simulink model "Final_EWASP_VC"  (R2022a)
settings: Solver=ode1  StartTime=0.0  StopTime=24*3600  FixedStep=10  RelTol=1e-3
values from neighbouring files (symbols this model uses):
  Aux_Threshold = 52    [Setup_Code_EWASP_VC.m]
  buildingAge = 2005    [Setup_Code_EWASP_VC.m]
  ceilingHeight = 2.4    [Setup_Code_EWASP_VC.m]
  conductiveHconnectMatrix = [ ... (first row only)    [Setup_Code_EWASP_VC.m]
  cRoofGreen = 100000    [Setup_Code_EWASP_VC.m]
  Defrost_After_Time = 30    [Setup_Code_EWASP_VC.m]
  DHWDemandProfile = occFreegainHotwaterElecTestPassiveOcc3(:,3)    [Setup_Code_EWASP_VC.m]
  Elec_Max = Elec_Max*(30/24.2)    [Setup_Code_EWASP_VC.m]
  Elec_Mid = Elec_Mid*(30/24.2)    [Setup_Code_EWASP_VC.m]
  Elec_Min = Elec_Min*(30/24.2)    [Setup_Code_EWASP_VC.m]
  ElecDemandProfile = occFreegainHotwaterElecTestPassiveOcc3(:,4)    [Setup_Code_EWASP_VC.m]
  ElecFixed = [Elec_Max(6,2) Elec_Max(6,4) Elec_Max(6,6) Elec_Max(6,7) ... (first row only)    [Setup_Code_EWASP_VC.m]
  floorOrCeilingArea = floorOrCeilingArea*1.15    [Setup_Code_EWASP_VC.m]
  forceCold = 0    [Setup_Code_EWASP_VC.m]
  freegain = occFreegainHotwaterElecTestPassiveOcc3(:,2)-max(occupancy)*25    [Setup_Code_EWASP_VC.m]
  furnitureModelOn = 1    [Setup_Code_EWASP_VC.m]
  Heat_Max = Heat_Max*(30/24.2)    [Setup_Code_EWASP_VC.m]
  Heat_Mid = Heat_Mid*(30/24.2)    [Setup_Code_EWASP_VC.m]
  Heat_Min = Heat_Min*(30/24.2)    [Setup_Code_EWASP_VC.m]
  HeatFixed = [Heat_Max(6,2) Heat_Max(6,4) Heat_Max(6,6) Heat_Max(6,7) ... (first row only)    [Setup_Code_EWASP_VC.m]
  HeatingOnProfile = repmat(HeatingOnProfile,365,1)    [Setup_Code_EWASP_VC.m]
  HEX_ReturnLowerLimit = 52.5    [Setup_Code_EWASP_VC.m]
  HEX_ReturnUpperLimit = 55    [Setup_Code_EWASP_VC.m]
  LeakMultiplier = 1+(2*(rand()-0.5)/10)    [Setup_Code_EWASP_VC.m]
  loopCap = 15    [Setup_Code_EWASP_VC.m]
  maxOcc = max(occupancyProfile)    [Setup_Code_EWASP_VC.m]
  NESW_wallArea = max(NESW_Lengths*ceilingHeight-NESW_Windows,0)    [Setup_Code_EWASP_VC.m]
  NESW_Windows = [ ... (first row only)    [Setup_Code_EWASP_VC.m]
  numRooms = roomCount    [Setup_Code_EWASP_VC.m]
  offsetDays = 0    [Setup_Code_EWASP_VC.m]
  pumpChoice = pumpChoices(MinIndex,1)    [Setup_Code_EWASP_VC.m]
  pumpRamp = 180    [Setup_Code_EWASP_VC.m]
  ReturnLowerLimit = 37.5    [Setup_Code_EWASP_VC.m]
  ReturnUpperLimit = 40    [Setup_Code_EWASP_VC.m]
  RoofIrradiance = Flat_NS_EW_RoofIrradiance(:,1)    [Setup_Code_EWASP_VC.m]
  roofStartTemp = ones(11,1)*20    [Setup_Code_EWASP_VC.m]
  rooftype = 0    [Setup_Code_EWASP_VC.m]
  RoomDataMatrix = [zeros(1,12);ones(1,12)*wallDensity;zeros(1,12);ones(1,12)*wallU;ones(1,12)*windowU;ones(1,12)*floorU;ones(1,12)*ceilingU;zeros(1,12);windowArea, 0;floorOrCeilingArea;zeros(1,12);floorOrCeilingArea*ceilingHeight]    [Setup_Code_EWASP_VC.m]
  roomVol = roomVol*1.15    [Setup_Code_EWASP_VC.m]
  slabStartTemp = (GroundTempTimeSeries(offsetDays*1440+1,1)+thermostatSetting)/2    [Setup_Code_EWASP_VC.m]
  SlackRequest = zeros(1440,1)    [Setup_Code_EWASP_VC.m]
  SolarThermalExists = 0    [Setup_Code_EWASP_VC.m]
  SourceFixed = HeatFixed-ElecFixed    [Setup_Code_EWASP_VC.m]
  StateSeries = StateSeriesGenerator(22,7,1)    [Setup_Code_EWASP_VC.m]
  Tank_Lower_Temp = 49.5    [Setup_Code_EWASP_VC.m]
  Tank_Upper_Temp = 52    [Setup_Code_EWASP_VC.m]
  Tank_Volume_m3 = 0.15    [Setup_Code_EWASP_VC.m]
  TankHeatHour = randi([1 5])-1    [Setup_Code_EWASP_VC.m]
  thermostatSetting = 20.0    (= 20)    [Setup_Code_EWASP_VC.m]
  upDown = [0;0;0;0;1;1;1;1;1;1;1]    [Setup_Code_EWASP_VC.m]
  variableASHP = 1    [Setup_Code_EWASP_VC.m]
  wallStartTempExt = thermostatSetting*(0.266+0.00215*outdoorStartTemp+0.018*wallU+0.00113*outdoorStartTemp*wallU+0.0068*wallU^2)    [Setup_Code_EWASP_VC.m]
undefined symbols (not defined in the file or in its folder): a, ceilingU, condUDMatrix, convUDMatrix, deltaPEXPANDED_E, deltaPEXPANDED_E2, deltaPEXPANDED_N, deltaPEXPANDED_N2, deltaPEXPANDED_S, deltaPEXPANDED_S2, deltaPEXPANDED_W, deltaPEXPANDED_W2, DesiredDHWTemp, DesiredFlowTempVsInOutDeltaTemp, DiffuseHorizontal, DiscIntNeverNeededParam, DNI, dwnAndConcrete, DWORK_A_HX, DWORK_CHK_FLU, DWORK_CP_NODE, DWORK_DH, DWORK_FLUID, DWORK_HCON, DWORK_LOSS, DWORK_MDOTDOWN, DWORK_MDOTIN, DWORK_MDOTUP, DWORK_MIX, DWORK_PRESS, DWORK_QDOTIN, DWORK_RHO_NODE, DWORK_TIN, DWORK_TS_OLD, DWORK_V_NODE, GroundTempTimeSeries, HCM, HCM2, HCM_closed, HCM_closed2, intermediateU, IsTop, massFlowMatrix, neighbourMatrix, numericalRoomUse, RadiatorMatrix, room2roomflowmatrix_E, room2roomflowmatrix_E2, room2roomflowmatrix_N, room2roomflowmatrix_N2, room2roomflowmatrix_S, room2roomflowmatrix_S2, room2roomflowmatrix_W, room2roomflowmatrix_W2, StateAirInEXPANDED_E, StateAirInEXPANDED_E2, StateAirInEXPANDED_N, StateAirInEXPANDED_N2, StateAirInEXPANDED_S, StateAirInEXPANDED_S2 ... (+23)
libraries: simulink x6, dspsigops x4, dspmtrx3 x4, carnot x3, spsEdgeDetectorLib x2, dspstat3 x2, powerlib_meascontrol x1, simulink_extras x1
(part 4 of 27)

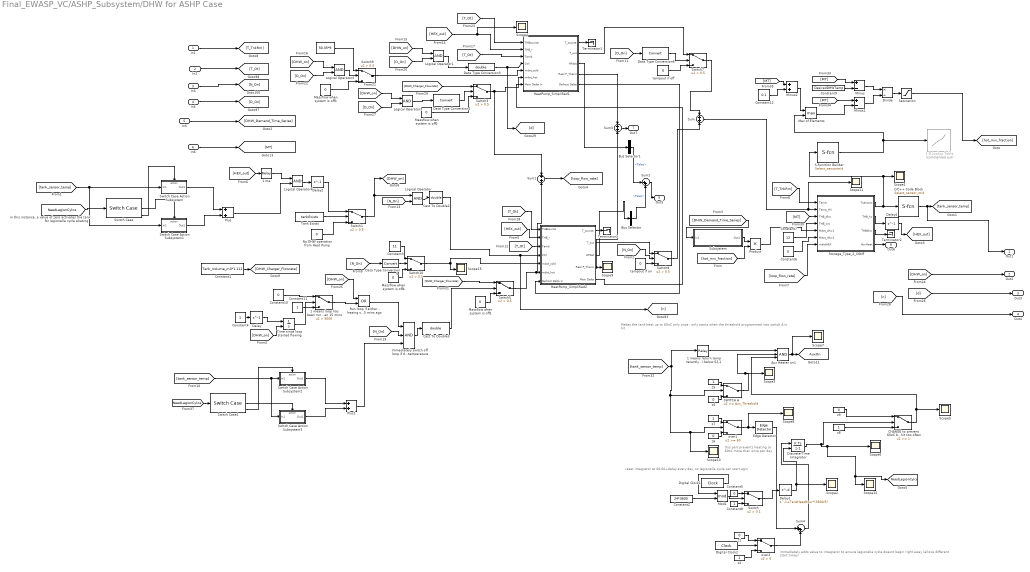
== system Final_EWASP_VC/ASHP_Subsystem/DHW for ASHP Case ==
  note: immediately adds value to integrator to ensure legionella cycle doesnt begin right away (allows different start times)
  note: this part prevents heating
      | to 60oC more than once per
      | day
  note: reset integrator at 00:00+delay every day,
      | so legionella cycle can start agin
  note: Makes the tank heat up to 60oC only once - only starts when the threshold programmed into switch A is hit
  In1 : Inport
  In2 : Inport  Port=2
  In3 : Inport  Port=3
  In4 : Inport  Port=4
  In5 : Inport  Port=5
  In6 : Inport  Port=6
  " " : Constant  Value=50.35*9  OutDataTypeStr=double
  1 me : Relay  OnSwitchValue=HEX_ReturnUpperLimit  OffSwitchValue=HEX_ReturnLowerLimit  OnOutputValue=0  OffOutputValue=1  OutDataTypeStr=boolean
  1 means loop has been running for less than 15 mins : Switch  Criteria=u2 > Threshold  Threshold=9000  SaturateOnIntegerOverflow=off  InputSameDT=off
  1 means return temp recently fell below 52.1 : Relay  OnSwitchValue=61  OffSwitchValue=59  OnOutputValue=0  OffOutputValue=1  OutDataTypeStr=boolean
  1-D Lookup Table : Lookup_n-D  Commented=on  NumberOfTableDimensions=1  BreakpointsForDimension1=[0:100]  Table="[1 1\t1\t1\t1\t1\t1\t1\t1\t1\t1\t1\t1\t1\t1\t1\t1\t1\t1\t1\t1\t1\t1\t1\t1\t1\t1\t1\t1\t1\t1\t1\t1\t1\t1\t1\t1\t1\t1\t1\t1\t1\t1\t1\t1\t1\t1\t1\t1\t1\t1\t1\t0.975000000000000\t0.951219512195122\t0.928571428571429\t0.906976744186047\t0.886363636363636\t0.866666666666667\t0.847826086956522\t0.829787234042553\t0.812500000000000\t0.795918367346939\t0.780000000000000\t0.764705882352941\t0.750000000000000\t0.735849056603774\t0.722222222222222\t0.709090909090909\t0.696428571428571\t0.684210526315790\t0.672413793103448\t0.661016949152542\t0.650000000000000\t0.639344262295082\t0.629032258064516\t0.619047619047619\t0.609375000000000\t0.600000000000000\t0.590909090909091\t0.582089552238806\t0.573529411764706\t0.565217391304348\t0.557142857142857\t0.549295774647887\t0.541666666666667\t0.534246575342466\t0.527027027027027\t0.520000000000000\t0.513157894736842\t0.506493506493506\t0.500000000000000\t0.493670886075949\t0.487500000000000\t0.481481481481481\t0.475609756097561\t0.469879518072289\t0.464285714285714\t0.458823529411765\t0.453488372093023\t0.448275862068966\t0.443181818181818]"  InternalRulePriority=Speed  RndMeth=Simplest
  Aux Heater on1 : Logic  Inputs=3  AllPortsSameDT=off  OutDataTypeStr=boolean
  Bus Selector : BusSelector  OutputSignals=Pelec
  Bus Selector1 : BusSelector  OutputSignals=Pelec
  C/C++ Code Block : S-Function  InitFcn=try, set_param(gcb,'FunctionName','Select_sensor_mid'), end  FunctionName=Select_sensor_mid  SFunctionModules=Select_sensor_mid_wrapper  SFunctionDeploymentMode=off  EnableBusSupport=off  mask(S-Function Builder){}
      mask help: Simulink:masks:SFunctionBuilder_MD
      mask init:
      | val = [[.9  0.75 0.75 1 1 .9 .9 1]',[1 1 0.75 0.75 .9 .9 1 .9]'];try , sys = get_param(gcb,'SfunBuilderFcnName');if isempty(sys), sys = get_param(gcb,'FunctionName'); end,catch, sys = get_param(gcb,'FunctionName'); end
      settings: CopyFcn=set_param(gcbh,'LinkStatus','none')  PreSaveFcn=try, set_param(gcb,'FunctionName','Select_sensor_mid'), end  OpenFcn=sfunctionwizard(gcbh)
      mask Display: plot(val(:,1),val(:,2)),disp(sys), port_label('input',1,'u0'), port_label('output',1,'y0')
  CHANGE to prevent 60oC being hit too often : Switch  Threshold=1  SaturateOnIntegerOverflow=off  InputSameDT=off
  Cast To Double2 : DataTypeConversion  OutDataTypeStr=double  SaturateOnIntegerOverflow=off  RndMeth=Floor
  Cast To Double3 : DataTypeConversion  OutDataTypeStr=double  SaturateOnIntegerOverflow=off  RndMeth=Floor
  Constant1 : Constant  Value=Tank_Volume_m3*1.111
  Constant10 : Constant  Value=0
  Constant11 : Constant
  Constant12 : Constant  Value=0.1
  Constant2 : Constant  Value=24*3600
  Constant3 : Constant  Value=11
  Constant4 : Constant
  Constant5 : Constant  Value=0
  Constant6 : Constant  Value=0
  Constant7 : Constant  Value=12
  Constant8 : Constant
  Constant9 : Constant  Value=DesiredDHWTemp
  Data Type Conversion3 : DataTypeConversion  OutDataTypeStr=double  SaturateOnIntegerOverflow=off  RndMeth=Floor
  Data Type Conversion4 : DataTypeConversion  RndMeth=Round  SaturateOnIntegerOverflow=off
  Data Type Conversion5 : DataTypeConversion  RndMeth=Round  SaturateOnIntegerOverflow=off
  Data Type Conversion6 : DataTypeConversion  RndMeth=Round  SaturateOnIntegerOverflow=off
  Delay : Delay  DelayLength=1  InitialCondition=0
  Delay1 : Delay  DelayLength=1+TankHeatHour*(3600/5)  InitialCondition=0
  Delay2 : Delay  DelayLength=1  InitialCondition=1
  Delay4 : Delay  DelayLength=1  InitialCondition=0
  Digital Clock1 : DigitalClock  SampleTime=10
  Digital Clock2 : DigitalClock  SampleTime=10
  Discrete-Time Integrator : DiscreteIntegrator  ExternalReset=rising  SampleTime=-1  OutDataTypeStr=double  ICPrevOutput=DiscIntNeverNeededParam  ICPrevScaledInput=DiscIntNeverNeededParam
  Divide : Product  Inputs=*/
  Edge Detector : spsEdgeDetectorLib/Edge Detector  model=Rising  ic=0  Ts=-1
      settings: SourceProductBaseCode=PS
  HeatPump_Simplified1 : Subsystem  AncestorBlock=carnot/Source/Heat_Pump/HeatPump  mask(heat pump){Tcin=[-5 15], Thout=[35 45 55 60], Qdotc=[-6125 -6125 -6125 -6125;-6125 -6125 -6125 -6125], Qdoth=[-3000*a -3000*a -3000*a -3000*a;-3000*a -3000*a -3000*a -3000*a], Pel=[1625*a 1625*a 1625*a 1625*a;1625*a 1625*a 1625*a 1625*a], caph=10*4180, capc=inf, UA=0, linc=10, quac=10, linh=10, quah=10}
      mask prompts: Tcin "inlet source temperature vector (°C)"; Thout "outlet load temperature vector (°C)"; Qdotc "source power matrix (W)"; Qdoth "heating power matrix (W)"; Pel "electric power matrix (W)"; caph "thermal capacity hot loop [J/K]"; capc "thermal capacity cold loop [J/K]"; UA "heat loss coefficient [W/K]"; linc "Cold side linear massflow dependant pressure drop in [Pa*s/kg]"; quac "Cold side quadratic massflow dependant pressure drop hot side in [Pa*s²/kg]"; linh "Hot side linear massflow dependant pressure drop in [Pa*s/kg]"; quah "Hot side quadratic massflow dependant pressure drop hot side in [Pa*s²/kg]"
      mask help:
      | Linearized heat pump model. Uses measured data according to EN 14511 as input.
      | heating power: Qdot_h = K1*Tcold_in + K2*Thot_out + K3
      | electric power: Pel = K4*Tcold_in + K5*Thot_out + K6
      | source power: Qdot_c = -K7*Tcold_in - K8*Thot_out - K9
      | differential equation: cap*dTh/dt = Qdot + mdot*cp*(T_in-T) + UA*(Tamb-T)
      | with: cap = mass * heat_capactiy
      | See hp_param.m for the parameters K1 to K9.
      | Literature: Schwamberger, K.: Fortschrittsberichete VDI, Nr. 263, 1991
      mask init:
      | % Matrix construction for hp_param
      | A = reshape(Qdoth',numel(Qdoth),1);
      | A = [A reshape(Qdotc',numel(Qdotc),1)];
      | A = [A reshape(Pel',numel(Pel),1)];
      | Thout_temp = [];
      | Tcin_temp = [];
      | for i=1:numel(Tcin)
      |     for j=1:numel(Thout)
      |         Tcin_temp = [Tcin_temp ; Tcin(i)];
      |     end
      |     Thout_temp = [Thout_temp ; Thout'];
      | end
      | A = [A Tcin_temp Thout_temp];
      | 
      | K = hp_param(A);
      | caph = max(1,caph);
      | capc = max(1,capc);
      mask Help: web(fullfile(path_carnot('help'),'heatpump.html'),'-helpbrowser')
      mask DialogControl ParameterTabVar0 Prompt: HP Caracteristic
      mask DialogControl ParameterTabVar01 Prompt: Thermal
      mask DialogControl ParameterTabVar012 Prompt: Hydraulic
      mask Display: plot(-20,-10,120,110,[10,20,40,60,80,90,90,80,60,40,20,10,10],[60,80,90,90,80,60,40,20,10,10,20,40,60],[40,20],[90,20],[60,80],[90,20],[50,50],[30,50],[60,40],[40,40],[57,43],[33,46],[44,57],[34,46])
  HeatPump_Simplified2 : Subsystem  AncestorBlock=carnot/Source/Heat_Pump/HeatPump  mask(heat pump){Tcin=[-5 5 12], Thout=[35 45 55 60], Qdotc=[4400*a-2000*a 4200*a-2000*a 3200*a-2000*a 1800*a-2000*a;5800*a-2100*a 5500*a-2100*a 4200*a-2100*a 2800*a-2100*a;8400*a-2200*a 7200*a-2200*a 5500*a-2200*a 3300*a-2200*a], Qdoth=[4400*a 4200*a 3200*a 1800*a;5800*a 5500*a 4200*a 2800*a;8400*a 7200*a 5500*a 3300*a], Pel=[2000*a 2000*a 2000*a 2000*a;2100*a 2100*a 2100*a 2100*a;2200*a 2200*a 2200*a 2200*a], caph=10*4180, capc=inf, UA=2, linc=10, quac=10, linh=10, quah=10}
      mask prompts: Tcin "inlet source temperature vector (°C)"; Thout "outlet load temperature vector (°C)"; Qdotc "source power matrix (W)"; Qdoth "heating power matrix (W)"; Pel "electric power matrix (W)"; caph "thermal capacity hot loop [J/K]"; capc "thermal capacity cold loop [J/K]"; UA "heat loss coefficient [W/K]"; linc "Cold side linear massflow dependant pressure drop in [Pa*s/kg]"; quac "Cold side quadratic massflow dependant pressure drop hot side in [Pa*s²/kg]"; linh "Hot side linear massflow dependant pressure drop in [Pa*s/kg]"; quah "Hot side quadratic massflow dependant pressure drop hot side in [Pa*s²/kg]"
      mask help:
      | Linearized heat pump model. Uses measured data according to EN 14511 as input.
      | heating power: Qdot_h = K1*Tcold_in + K2*Thot_out + K3
      | electric power: Pel = K4*Tcold_in + K5*Thot_out + K6
      | source power: Qdot_c = -K7*Tcold_in - K8*Thot_out - K9
      | differential equation: cap*dTh/dt = Qdot + mdot*cp*(T_in-T) + UA*(Tamb-T)
      | with: cap = mass * heat_capactiy
      | See hp_param.m for the parameters K1 to K9.
      | Literature: Schwamberger, K.: Fortschrittsberichete VDI, Nr. 263, 1991
      mask init: same as Final_EWASP_VC/ASHP_Subsystem/DHW for ASHP Case/HeatPump_Simplified1
      mask Help: web(fullfile(path_carnot('help'),'heatpump.html'),'-helpbrowser')
      mask DialogControl ParameterTabVar0 Prompt: HP Caracteristic
      mask DialogControl ParameterTabVar01 Prompt: Thermal
      mask DialogControl ParameterTabVar012 Prompt: Hydraulic
      mask Display: plot(-20,-10,120,110,[10,20,40,60,80,90,90,80,60,40,20,10,10],[60,80,90,90,80,60,40,20,10,10,20,40,60],[40,20],[90,20],[60,80],[90,20],[50,50],[30,50],[60,40],[40,40],[57,43],[33,46],[44,57],[34,46])
  "Immediately switch off loop if defrost is required, or if tank reaches temperature" : Logic  Inputs=3  AllPortsSameDT=off  OutDataTypeStr=boolean
  Logical Operator{,1..4} (5 alike) : Logic  AllPortsSameDT=off  OutDataTypeStr=boolean
  Massflow when system is off{1..4} (4 alike) : Constant  Value=0
  Max of Elements : MinMax  Function=max  Inputs=2
  Minus : Sum  Inputs=+-
  Minus1 : Sum  Inputs=+-
  Minus2 : Sum  Inputs=2
  Mod1 : Math  Operator=mod  SignedPower=on
  No DHW operation from Heat Pump : Constant  Value=0
  Plus : Sum
  Plus1 : Sum
  Product : Product
  "Run loop if either - heaing system is on, heating system was activated less than 15 mins ago" : Logic  Operator=OR  AllPortsSameDT=off  OutDataTypeStr=boolean
  S-Function Builder : S-Function  InitFcn=try, set_param(gcb,'FunctionName','Select_sensor'), end  FunctionName=Select_sensormid  SFunctionModules=Select_sensor_wrapper  SFunctionDeploymentMode=off  EnableBusSupport=off  mask(S-Function Builder){}
      mask help: Simulink:masks:SFunctionBuilder_MD
      mask init: same as Final_EWASP_VC/ASHP_Subsystem/DHW for ASHP Case/C/C++ Code Block
      settings: CopyFcn=set_param(gcbh,'LinkStatus','none')  PreSaveFcn=try, set_param(gcb,'FunctionName','Select_sensormid'), end  OpenFcn=sfunctionwizard(gcbh)
      mask Display: plot(val(:,1),val(:,2)),disp(sys), port_label('input',1,'u0'), port_label('output',1,'y0')
  SWITCH A : Switch  Threshold=Aux_Threshold  SaturateOnIntegerOverflow=off  InputSameDT=off
  Saturation : Saturate  UpperLimit=1  LowerLimit=0
  Scope{1..12,15} (13 alike) : Scope
  Storage_Type_2_CONF : Subsystem  AncestorBlock=carnot/Storage/Thermal/Storage_Type_2_CONF  mask(Storage for hot water production){t0=52.1, hgt=1.5279, stgtype=2, tini=[52.1 52.1 52.1 52.1 52.1 52.1 52.1 52.1 52.1 52.1], mpts=[1 2 3 4 5 6 7 8 9 10], PathName=fullfile(pwd,'TankVolTemp'), FileName='<user defined>', userPath=on, userParam=on, uwall=0.235, ubot=0.235, utop=0.235, axcond=0.235, volume=Tank_Volume_m3, dia=((4/(3*3.142))*Tank_Volume_m3)^(1/3), standing=standing cylinder, nodes=10, mpoints=10, Tsensor=[0.1:0.1:0.9], hx1inlet=0.45, hx1outlet=0, hx1dia=0.03, hx1uac=500, hx1uam=0.15, hx1uat=0.6, hx1dpqua=20, hx1dplin=20, pipe1inlet=0, pipe1outlet=1, pipe1dia=0.03, pipe2inlet=0.6, pipe2outlet=1, pipe2dia=0.03}
      mask prompts: t0 "Initial temperature (vector or scalar) in °C"; hgt "Height of storage in m"; stgtype "Storage Type (0..5)"; tini "Start temperatures of nodes in °C"; mpts "Index to measured nodes"; PathName "Path"; FileName "Parameter set"; userPath "Edit path and name of parameter set"; userParam "User defined parameters"; uwall "Heat transfer coefficient to ambient [W/m²K]"; ubot "Heat transfer coefficient to ambient bottom [W/m²K]"; utop "Heat transfer coefficient to ambient top [W/m²K]"; axcond "Effective thermal conductivity [W/m/K]"; volume "Volume [m³]"; dia "Diameter [m]"; standing "Position"; nodes "Number of nodes"; mpoints "Number of node temperatures (for display)"; Tsensor "Temperature sensor position (0..1, 0 = bottom, 1 = top)"; hx1inlet "relative height of inlet"; hx1outlet "relative height of outlet"; hx1dia "Diameter of HX pipe [m]"; hx1uac "uac: heat transfer coefficient [W/K /(kg/s) /(°C)]"; hx1uam "uam: massflow dependent heat transfer [-]"; hx1uat "uat: temperature difference dependent heat transfer [-]"; hx1dpqua "pressure drop quadratic in mdot [Pa*s²/kg²]"; hx1dplin "pressure drop linear in mdot [Pa*s/kg]"; pipe1inlet "relative height of inlet, range from 0 (= bottom) to 1 (= top)"; pipe1outlet "relative height of outlet, range from 0 (= bottom) to 1 (= top)"; pipe1dia "Diameter of pipe in m"; pipe2inlet "relative height of inlet, range from 0 (= bottom) to 1 (= top)"; pipe2outlet "relative height of outlet, range from 0 (= bottom) to 1 (= top)"; pipe2dia "Diameter of pipe in m"
      mask help:
      | Storage for hot water production (domestic hot water cylinder). The storage model has the following components (with their typical position):
      | - one charging heat exchanger (lower part)
      | - one pipe connection for the hot water (total height)
      | - one pipe connection for the hot water circulation (upper part )
      mask init:
      | %[ok, param] = CarnotCallbacks_StorageConf('SetParam',stgtype,gcbh,PathName,FileName);
      mask Help: web(fullfile(path_carnot('help'),'Storage_Type_N.html'),'-helpbrowser')
      mask TypeOptions hgt: HX_EN12977_1/hgt | Pipe_Connection_1/hgt | Pipe_Connection_2/hgt
      mask TypeOptions stgtype: CreateSdat/stgtype
      mask TypeOptions tini: sfun_storageTnodesjh/tini
      mask TypeOptions mpts: select_T/Indices
      mask Callback userPath: [ok, param] = CarnotCallbacks_StorageConf('UserEdit',2,gcbh);
      mask Callback userParam: [ok, param] = CarnotCallbacks_StorageConf('UserEdit',2,gcbh);
      mask TypeOptions uwall: sfun_storageTnodesjh/uloss
      mask TypeOptions ubot: sfun_storageTnodesjh/ubot
      mask TypeOptions utop: sfun_storageTnodesjh/utop
      mask TypeOptions axcond: sfun_storageTnodesjh/cond
      mask TypeOptions volume: sfun_storageTnodesjh/volume
      mask TypeOptions dia: sfun_storageTnodesjh/dia
      mask TypeOptions standing: sfun_storageTnodesjh/standing
      mask TypeOptions nodes: sfun_storageTnodesjh/nodes | select_T/InputPortWidth | HX_EN12977_1/nodes | HX_EN12977_2/nodes | HX_EN12977_3/nodes | Pipe_Connection_1/nodes | Pipe_Connection_2/nodes | Pipe_Connection_3/nodes
      mask TypeOptions Tsensor: T_Sensor_Surface/pos
      mask TypeOptions hx1inlet: HX_EN12977_1/h_in
      mask TypeOptions hx1outlet: HX_EN12977_1/h_out
      mask TypeOptions hx1dia: HX_EN12977_1/dia
      mask TypeOptions hx1uac: HX_EN12977_1/ua0
      mask TypeOptions hx1uam: HX_EN12977_1/uam
      mask TypeOptions hx1uat: HX_EN12977_1/uat
      mask TypeOptions hx1dpqua: HX_EN12977_1/dpqua
      mask TypeOptions hx1dplin: HX_EN12977_1/dplin
      mask TypeOptions pipe1inlet: Pipe_Connection_1/h_in
      mask TypeOptions pipe1outlet: Pipe_Connection_1/h_out
      mask TypeOptions pipe1dia: Pipe_Connection_1/dia
      mask TypeOptions pipe2inlet: Pipe_Connection_2/h_in
      mask TypeOptions pipe2outlet: Pipe_Connection_2/h_out
      mask TypeOptions pipe2dia: Pipe_Connection_2/dia
      mask DialogControl Container14 Prompt: Infos
      mask DialogControl ParameterGroupVar Prompt: Picking a parameter set
      mask DialogControl Control3 Prompt: Carnot public data
      mask DialogControl Control3 Callback: [ok, file] = CarnotCallbacks_StorageConf('GetFilename',2,gcbh,'public');
      mask DialogControl Control4 Prompt: Carnot internal data
      mask DialogControl Control4 Callback: [ok, file] = CarnotCallbacks_StorageConf('GetFilename',2,gcbh,'internal');
      mask DialogControl Control2 Prompt: Selected path
      mask DialogControl Control2 Callback: [ok, file] = CarnotCallbacks_StorageConf('GetFilename',2,gcbh,'selected');
      mask DialogControl Container4 Prompt: Parameter values
      mask DialogControl Container6 Prompt: Storage
      mask DialogControl Container8 Prompt: Connections
      mask DialogControl Container11 Prompt: Heat exchanger
      mask DialogControl Container9 Prompt: Discharging pipe
      mask DialogControl Container12 Prompt: Circulation pipe
      mask DialogControl Control6 Prompt: Save in Carnot internal data
      mask DialogControl Control6 Callback: [ok, param] = CarnotCallbacks_StorageConf('SaveFilename',2,gcbh,'internal','STG');
      mask DialogControl Control5 Prompt: Save in selected path
      mask DialogControl Control5 Callback: [ok, param] = CarnotCallbacks_StorageConf('SaveFilename',2,gcbh,'selected','STG');
      mask Display:
      | % user defined picture file
      | namestr = ['Storage_Type_', num2str(get_param(gcb,'stgtype'))];
      | picfile = fullfile(path_carnot('intlibsl'), 'Storage','Thermal', ...
      |     namestr,'parameter_set', [namestr, '.jpg']);
      | 
      | % show public picture
      | plot([36,36,40,50,54,54,50,40,36]/90,...
      |     [90,50,45,45,50,90,93,93,90]/100,[36,51,44,51,36]/90,...
      |     [50,50,55,60,60]/100)
      | set_param(gcb, 'BackgroundColor', 'Red')
      | 
      | % show internal picture if defined
      | if  ~BlockIsInCarnotLibrary       % if not located in library
      |     if exist(picfile, 'file')
      |         image(imread(picfile), [0.25, 0, 0.45, 1])
      |         set_param(gcb, 'BackgroundColor', 'White')
      |     end
      | end
  Subsystem : Subsystem
      mask Display:
      | disp('Minute to \n Second Res')
      | port_label('input', 1, 'min res')
      | port_label('output', 1, 'sec res')
  Sum : Sum
  Sum1 : Sum
  Sum2 : Sum  Inputs=|++
  Sum3 : Sum
  Sum4 : Sum  Inputs=|++
  Switch : Switch  Criteria=u2 > Threshold  Threshold=0.1  SaturateOnIntegerOverflow=off  InputSameDT=off
  Switch Case : SwitchCase  CaseConditions={1,0}
  Switch Case Action Subsystem : Subsystem  TreatAsAtomicUnit=on
  Switch Case Action Subsystem1 : Subsystem  TreatAsAtomicUnit=on
  Switch Case Action Subsystem2 : Subsystem  TreatAsAtomicUnit=on
  Switch Case Action Subsystem3 : Subsystem  TreatAsAtomicUnit=on
  Switch Case1 : SwitchCase  CaseConditions={1,0}
  Switch{1,3,5,7..10} (7 alike) : Switch  Criteria=u2 > Threshold  Threshold=0.5  SaturateOnIntegerOverflow=off  InputSameDT=off
  Tank Exists : Constant  Value=tankExists
  Terminator1 : Terminator
  Terminator2 : Terminator
  Terminator3 : Terminator
  Time since loop started flowing : Integrator  ExternalReset=rising
  over1 : Switch  Threshold=60  SaturateOnIntegerOverflow=off  InputSameDT=off
  over2 : Switch  Criteria=u2 > Threshold  SaturateOnIntegerOverflow=off  InputSameDT=off
  tempout if off : Constant  Value=0
  tempout if on : Constant  Value=0
  z{1,4,6,9} (4 alike) : Constant  Value=0
  z{2,5,7..8} (4 alike) : Constant
  Out1 : Outport  VectorParamsAs1DForOutWhenUnconnected=off
  Out2 : Outport  Port=2  VectorParamsAs1DForOutWhenUnconnected=off
  Out3 : Outport  Port=3  VectorParamsAs1DForOutWhenUnconnected=off
  Out4 : Outport  Port=4  VectorParamsAs1DForOutWhenUnconnected=off
  Out5 : Outport  Port=5  VectorParamsAs1DForOutWhenUnconnected=off
  Out6 : Outport  Port=6  VectorParamsAs1DForOutWhenUnconnected=off
  Out7 : Outport  Port=7  VectorParamsAs1DForOutWhenUnconnected=off
  tag scope: AuxOn=global, NeedLegionCylce=global
  wires:
  [T_Ot] -> HeatPump_Simplified2/3(Tamb)
  [DHW_Charger_Flowrate] -> Switch5/1
  [HEX_out] -> Scope4/1, HeatPump_Simplified1/2(THB_r)
  [T_Ot] -> HeatPump_Simplified1/3(Tamb)
  In4/1 -> [D_On]
  Logical Operator1/1 -> Data Type Conversion3/1
  [T_TnkRm] -> Storage_Type_2_CONF/1(Tamb)
  Sum1/1 -> [loop_flow_rate]
  Product/1 -> Storage_Type_2_CONF/5(Mdot_dhw1)
  "Immediately switch off loop if defrost is required, or if tank reaches temperature"/1 -> Cast To Double3/1
  [DHW_on] -> "Run loop if either - heaing system is on, heating system was activated less than 15 mins ago"/1
  Constant11/1 -> 1 means loop has been running for less than 15 mins/3
  Switch8/1 -> Sum/2
  Constant7/1 -> Storage_Type_2_CONF/4(THB_circ)
  [DHW_Charger_Flowrate] -> Switch3/1
  " "/1 -> Switch9/1
  [DHW_on] -> Out2/1
  HeatPump_Simplified2/5(Main Delta) -> HeatPump_Simplified1/7(Main Delta In)
  Constant6/1 -> Storage_Type_2_CONF/6(Mdot_dhw2)
  In3/1 -> [N_On]
  Constant4/1 -> Delay/1
  Delay/1 -> Time since loop started flowing/1
  HeatPump_Simplified2/2("T_out ") -> Switch8/1
  HeatPump_Simplified1/1(T_source) -> Terminator1/1
  Storage_Type_2_CONF/1(Tsensors) -> S-Function Builder/1, Scope1/1, C/C++ Code Block/1
  Constant10/1 -> 1 means loop has been running for less than 15 mins/1
  "Run loop if either - heaing system is on, heating system was activated less than 15 mins ago"/1 -> "Immediately switch off loop if defrost is required, or if tank reaches temperature"/1
  Storage_Type_2_CONF/3(THBdhw) -> Terminator2/1
  Data Type Conversion3/1 -> [d], HeatPump_Simplified1/4(Ctrl)
  Sum/1 -> Scope11/1, Storage_Type_2_CONF/2(Temp_HX)
  Logical Operator/1 -> Cast To Double2/1
  [D_On] -> Data Type Conversion6/1
  tempout if off/1 -> Switch7/3
  Cast To Double3/1 -> Switch5/2
  Massflow when system is off4/1 -> Switch10/3
  Massflow when system is off1/1 -> Switch5/3
  In6/1 -> [MT]
  [tank_sensor_temp] -> Switch Case Action Subsystem1/1(In1), Switch Case Action Subsystem/1(In1)
  Cast To Double2/1 -> [n], HeatPump_Simplified2/4(Ctrl)
  HeatPump_Simplified1/2("T_out ") -> Switch7/1
  Data Type Conversion4/1 -> Switch3/2
  [DHW_on] -> Time since loop started flowing/2
  [hot_mix_fraction] -> Product/2
  HeatPump_Simplified2/1(T_source) -> Terminator3/1
  Logical Operator3/1 -> Data Type Conversion4/1
  [N_On] -> Logical Operator/2
  Switch Case Action Subsystem/1(Out1) -> Plus/1
  Delay4/1 -> [HEX_out]
  Data Type Conversion6/1 -> Switch7/2
  Switch10/1 -> HeatPump_Simplified2/5(mdot_cold), Scope15/1
  C/C++ Code Block/1 -> Out1/1, [tank_sensor_temp]
  [loop_flow_rate] -> Storage_Type_2_CONF/7(mdotHEX)
  Subsystem/1(Out1) -> Product/1
  1 me/1 -> Logical Operator4/1
  HeatPump_Simplified2/3(HPdat) -> Bus Selector/1
  [HEX_out] -> HeatPump_Simplified2/2(THB_r)
  [T_Ot] -> HeatPump_Simplified1/1(THBsource)
  [N_On] -> Data Type Conversion5/1
  [N_On] -> "Immediately switch off loop if defrost is required, or if tank reaches temperature"/2
  Massflow when system is off2/1 -> Switch3/3
  [T_Ot] -> HeatPump_Simplified2/1(THBsource)
  Data Type Conversion5/1 -> Switch10/2
  Logical Operator2/1 -> Switch9/2
  Switch5/1 -> Sum1/2, HeatPump_Simplified2/6(mdot_hot)
  HeatPump_Simplified2/4(Real P_Therm) -> Sum3/2, Scope9/1
  tempout if on/1 -> Switch8/3
  [N_On] -> Switch8/2
  Switch9/1 -> HeatPump_Simplified1/5(mdot_cold)
  1 means loop has been running for less than 15 mins/1 -> "Run loop if either - heaing system is on, heating system was activated less than 15 mins ago"/2
  Constant3/1 -> Switch10/1
  HeatPump_Simplified1/5(Defrost Delta) -> HeatPump_Simplified2/7(Defrost Delta In)
  Storage_Type_2_CONF/2(THB_hx) -> Delay4/1
  [DHW_Demand_Time_Series] -> Subsystem/1(In1)
  [d] -> Out3/1
  Switch7/1 -> Sum/1
  Switch3/1 -> Sum1/1, HeatPump_Simplified1/6(mdot_hot)
  Massflow when system is off3/1 -> Switch9/3
  [tank_sensor_temp] -> Switch Case Action Subsystem3/1(In1), Switch Case Action Subsystem2/1(In1)
  Time since loop started flowing/1 -> 1 means loop has been running for less than 15 mins/2
  HeatPump_Simplified1/4(Real P_Therm) -> Sum3/1
  [MT] -> Storage_Type_2_CONF/3(THB_dhw)
  In5/1 -> [DHW_Demand_Time_Series]
  In1/1 -> [T_TnkRm]
  In2/1 -> [T_Ot]
  [n] -> Out4/1
  [DHW_on] -> Logical Operator1/1
  [D_On] -> Logical Operator1/2
  [DHW_on] -> Logical Operator2/1
  [D_On] -> Logical Operator2/2
  [DHW_on] -> Logical Operator3/1
  [D_On] -> Logical Operator3/2
  Logical Operator4/1 -> Delay2/1
  Delay2/1 -> Switch1/1
  [HEX_out] -> 1 me/1
  z5/1 -> SWITCH A/1
  z4/1 -> SWITCH A/3
  SWITCH A/1 -> Scope3/1, Aux Heater on1/2
  1 means return temp recently fell below 52.1/1 -> Aux Heater on1/1
  Aux Heater on1/1 -> Scope7/1, [AuxOn]
  z6/1 -> over1/3
  z7/1 -> over1/1
  [tank_sensor_temp] -> 1 means return temp recently fell below 52.1/1, Scope10/1, over1/2, SWITCH A/2
  over1/1 -> Scope8/1, Edge Detector/1
  Edge Detector/1 -> Sum4/1
  z9/1 -> CHANGE to prevent 60oC being hit too often/1
  Discrete-Time Integrator/1 -> [NeedLegionCylce], Scope12/1, Scope6/1, CHANGE to prevent 60oC being hit too often/2
  z8/1 -> CHANGE to prevent 60oC being hit too often/3
  CHANGE to prevent 60oC being hit too often/1 -> Scope5/1, Aux Heater on1/3
  Constant1/1 -> [DHW_Charger_Flowrate]
  Digital Clock1/1 -> Mod1/1
  Constant5/1 -> Switch/1
  Mod1/1 -> Switch/2
  Constant2/1 -> Mod1/2
  Constant8/1 -> Switch/3
  Switch/1 -> Delay1/1
  [MT] -> Minus/1
  Constant9/1 -> Minus/2
  [MT] -> Minus1/1
  S-Function Builder/1 -> Max of Elements/2, 1-D Lookup Table/1
  Minus/1 -> Divide/1
  Minus1/1 -> Divide/2
  Divide/1 -> Saturation/1
  Max of Elements/1 -> Minus1/2
  [MT] -> Minus2/1
  Constant12/1 -> Minus2/2
  Minus2/1 -> Max of Elements/1
  Saturation/1 -> [hot_mix_fraction]
  Bus Selector/1 -> Sum2/2  "<Pelec>"
  Bus Selector1/1 -> Sum2/1  "<Pelec>"
  HeatPump_Simplified1/3(HPdat) -> Bus Selector1/1
  Sum2/1 -> Out5/1
  Storage_Type_2_CONF/4(AuxHeat) -> Out6/1
  Switch1/1 -> [DHW_on], Logical Operator/1
  Tank Exists/1 -> Switch1/2
  No DHW operation from Heat Pump/1 -> Switch1/3
  Sum3/1 -> Out7/1
  Delay1/1 -> Discrete-Time Integrator/2, Scope2/1
  z1/1 -> over2/1
  z2/1 -> over2/3
  Digital Clock2/1 -> over2/2
  over2/1 -> Sum4/2
  Sum4/1 -> Discrete-Time Integrator/1
  Switch Case/3 -> Switch Case Action Subsystem/Action
  Switch Case/2 -> Switch Case Action Subsystem1/Action
  Switch Case Action Subsystem1/1(Out1) -> Plus/2
  Plus/1 -> Logical Operator4/2
  [NeedLegionCylce] -> Switch Case/1
  [NeedLegionCylce] -> Switch Case1/1
  Switch Case1/3 -> Switch Case Action Subsystem2/Action
  Switch Case1/2 -> Switch Case Action Subsystem3/Action
  Switch Case Action Subsystem2/1(Out1) -> Plus1/1
  Switch Case Action Subsystem3/1(Out1) -> Plus1/2
  Plus1/1 -> "Immediately switch off loop if defrost is required, or if tank reaches temperature"/3

== system Final_EWASP_VC/ASHP_Subsystem/Defrost Timer ==
  In1 : Inport
  In2 : Inport  Port=2
  In3 : Inport  Port=3
  Add : Sum  Inputs=-
  Add1 : Sum
  Cast To Double : DataTypeConversion  OutDataTypeStr=double  SaturateOnIntegerOverflow=off  RndMeth=Floor
  Logical Operator : Logic  AllPortsSameDT=off  OutDataTypeStr=boolean
  Minus : Sum  Inputs=+-  SaturateOnIntegerOverflow=on
  NOT : Logic  Operator=NOT  IconShape=distinctive  AllPortsSameDT=off  OutDataTypeStr=boolean
  NOT1 : Logic  Operator=NOT  IconShape=distinctive  AllPortsSameDT=off  OutDataTypeStr=boolean
  NOT2 : Logic  Operator=NOT  IconShape=distinctive  AllPortsSameDT=off  OutDataTypeStr=boolean
  Saturation : Saturate  UpperLimit=1  LowerLimit=0
  Scope : Scope  NumInputPorts=3
  Scope1 : Scope  NumInputPorts=2
  Scope2 : Scope
  Scope3 : Scope
  Subsystem : Subsystem
  Subsystem1 : Subsystem
  Out1 : Outport  VectorParamsAs1DForOutWhenUnconnected=off
  Out2 : Outport  Port=2  VectorParamsAs1DForOutWhenUnconnected=off
  wires:
  Logical Operator/1 -> NOT1/1, Cast To Double/1
  Subsystem/3(Out3) -> Subsystem1/3(In3)
  Cast To Double/1 -> Add1/1
  NOT2/1 -> Out1/1
  Subsystem/2(Out2) -> Subsystem1/2(In2)
  NOT1/1 -> Scope/3, Minus/2
  Add1/1 -> NOT/1, Subsystem/2(In2)
  Subsystem1/1(Out1) -> Scope1/1, Add/1
  Subsystem/1(Out1) -> Scope2/1, Subsystem1/1(In1)
  In2/1 -> Logical Operator/1
  NOT/1 -> Scope/2, Minus/1
  Add/1 -> Scope1/2, Add1/2
  In1/1 -> Subsystem/1(In1)
  In3/1 -> Logical Operator/2
  Minus/1 -> Saturation/1
  Saturation/1 -> Scope3/1, Scope/1, Out2/1, NOT2/1

== system Final_EWASP_VC/ASHP_Subsystem/Subsystem14 ==
  In1 : Inport
  In2 : Inport  Port=2
  In3 : Inport  Port=3
  In4 : Inport  Port=4
  In5 : Inport  Port=5
  In6 : Inport  Port=6
  In7 : Inport  Port=7
  In8 : Inport  Port=8
  Add : Sum
  Based on 50.35l/s per kW (https://designbuilder.co.uk/helpv5.5/Content/AirToWaterHeatPumpASHPData.htm)1 : Constant  Value=50.35*9  OutDataTypeStr=double
  Based on 50.35l/s per kW (https://designbuilder.co.uk/helpv5.5/Content/AirToWaterHeatPumpASHPData.htm)2 : Constant  Value=50.35*9  OutDataTypeStr=double
  Bus Selector1 : BusSelector  OutputSignals=Pelec  OutputAsBus=on
  Bus Selector2 : BusSelector  OutputSignals=Pelec  OutputAsBus=on
  Data Type Conversion{2..3,8,10} (4 alike) : DataTypeConversion  OutDataTypeStr=double  SaturateOnIntegerOverflow=off  RndMeth=Floor
  Data Type Conversion{4..7} (4 alike) : DataTypeConversion  RndMeth=Round  SaturateOnIntegerOverflow=off
  Digital Clock : DigitalClock  SampleTime=10
  Digital Clock1 : DigitalClock  SampleTime=10
  Discrete-Time Integrator : DiscreteIntegrator  SampleTime=-1  ICPrevOutput=DiscIntNeverNeededParam  ICPrevScaledInput=DiscIntNeverNeededParam
  Ground1 : Ground
  HeatPump_Simplified : Subsystem  AncestorBlock=carnot/Source/Heat_Pump/HeatPump  mask(heat pump){Tcin=[-5 7 12], Thout=[35 45 55 60], Qdotc=[4400*a-2000*a 4200*a-2000*a 3200*a-2000*a 1800*a-2000*a;5800*a-2100*a 5500*a-2100*a 4200*a-2100*a 2800*a-2100*a;8400*a-2200*a 7200*a-2200*a 5500*a-2200*a 3300*a-2200*a], Qdoth=[4400*a 4200*a 3200*a 1800*a;5600*a 5500*a 4200*a 2800*a;8400*a 7200*a 5500*a 3300*a], Pel=[2000*a 2000*a 2000*a 2000*a;2100*a 2100*a 2100*a 2100*a;2200*a 2200*a 2200*a 2200*a], caph=loopCap*4180, capc=inf, UA=7, linc=10, quac=10, linh=10, quah=10}
      mask prompts: Tcin "inlet source temperature vector (°C)"; Thout "outlet load temperature vector (°C)"; Qdotc "source power matrix (W)"; Qdoth "heating power matrix (W)"; Pel "electric power matrix (W)"; caph "thermal capacity hot loop [J/K]"; capc "thermal capacity cold loop [J/K]"; UA "heat loss coefficient [W/K]"; linc "Cold side linear massflow dependant pressure drop in [Pa*s/kg]"; quac "Cold side quadratic massflow dependant pressure drop hot side in [Pa*s²/kg]"; linh "Hot side linear massflow dependant pressure drop in [Pa*s/kg]"; quah "Hot side quadratic massflow dependant pressure drop hot side in [Pa*s²/kg]"
      mask help:
      | Linearized heat pump model. Uses measured data according to EN 14511 as input.
      | heating power: Qdot_h = K1*Tcold_in + K2*Thot_out + K3
      | electric power: Pel = K4*Tcold_in + K5*Thot_out + K6
      | source power: Qdot_c = -K7*Tcold_in - K8*Thot_out - K9
      | differential equation: cap*dTh/dt = Qdot + mdot*cp*(T_in-T) + UA*(Tamb-T)
      | with: cap = mass * heat_capactiy
      | See hp_param.m for the parameters K1 to K9.
      | Literature: Schwamberger, K.: Fortschrittsberichete VDI, Nr. 263, 1991
      mask init: same as Final_EWASP_VC/ASHP_Subsystem/DHW for ASHP Case/HeatPump_Simplified1
      mask Help: web(fullfile(path_carnot('help'),'heatpump.html'),'-helpbrowser')
      mask DialogControl ParameterTabVar0 Prompt: HP Caracteristic
      mask DialogControl ParameterTabVar01 Prompt: Thermal
      mask DialogControl ParameterTabVar012 Prompt: Hydraulic
      mask Display: plot(-20,-10,120,110,[10,20,40,60,80,90,90,80,60,40,20,10,10],[60,80,90,90,80,60,40,20,10,10,20,40,60],[40,20],[90,20],[60,80],[90,20],[50,50],[30,50],[60,40],[40,40],[57,43],[33,46],[44,57],[34,46])
  HeatPump_Simplified1 : Subsystem  AncestorBlock=carnot/Source/Heat_Pump/HeatPump  mask(heat pump){Tcin=[-5 15], Thout=[35 45 55 60], Qdotc=[-6125 -6125 -6125 -6125;-6125 -6125 -6125 -6125], Qdoth=[-3000*a -3000*a -3000*a -3000*a;-3000*a -3000*a -3000*a -3000*a], Pel=[1625*a 1625*a 1625*a 1625*a;1625*a 1625*a 1625*a 1625*a], caph=loopCap*4180, capc=inf, UA=0, linc=10, quac=10, linh=10, quah=10}
      mask prompts: Tcin "inlet source temperature vector (°C)"; Thout "outlet load temperature vector (°C)"; Qdotc "source power matrix (W)"; Qdoth "heating power matrix (W)"; Pel "electric power matrix (W)"; caph "thermal capacity hot loop [J/K]"; capc "thermal capacity cold loop [J/K]"; UA "heat loss coefficient [W/K]"; linc "Cold side linear massflow dependant pressure drop in [Pa*s/kg]"; quac "Cold side quadratic massflow dependant pressure drop hot side in [Pa*s²/kg]"; linh "Hot side linear massflow dependant pressure drop in [Pa*s/kg]"; quah "Hot side quadratic massflow dependant pressure drop hot side in [Pa*s²/kg]"
      mask help:
      | Linearized heat pump model. Uses measured data according to EN 14511 as input.
      | heating power: Qdot_h = K1*Tcold_in + K2*Thot_out + K3
      | electric power: Pel = K4*Tcold_in + K5*Thot_out + K6
      | source power: Qdot_c = -K7*Tcold_in - K8*Thot_out - K9
      | differential equation: cap*dTh/dt = Qdot + mdot*cp*(T_in-T) + UA*(Tamb-T)
      | with: cap = mass * heat_capactiy
      | See hp_param.m for the parameters K1 to K9.
      | Literature: Schwamberger, K.: Fortschrittsberichete VDI, Nr. 263, 1991
      mask init: same as Final_EWASP_VC/ASHP_Subsystem/DHW for ASHP Case/HeatPump_Simplified1
      mask Help: web(fullfile(path_carnot('help'),'heatpump.html'),'-helpbrowser')
      mask DialogControl ParameterTabVar0 Prompt: HP Caracteristic
      mask DialogControl ParameterTabVar01 Prompt: Thermal
      mask DialogControl ParameterTabVar012 Prompt: Hydraulic
      mask Display: plot(-20,-10,120,110,[10,20,40,60,80,90,90,80,60,40,20,10,10],[60,80,90,90,80,60,40,20,10,10,20,40,60],[40,20],[90,20],[60,80],[90,20],[50,50],[30,50],[60,40],[40,40],[57,43],[33,46],[44,57],[34,46])
  Logical Operator{1..4} (4 alike) : Logic  AllPortsSameDT=off  OutDataTypeStr=boolean
  Logical Operator6 : Logic  Inputs=4  AllPortsSameDT=off  OutDataTypeStr=boolean
  Massflow when system is off{1..4} (4 alike) : Constant  Value=0
  Product3 : Product
  Product4 : Product
  Relay2 : Relay  OnSwitchValue=ReturnUpperLimit  OffSwitchValue=ReturnLowerLimit  OnOutputValue=0  OffOutputValue=1  OutDataTypeStr=boolean
  Scope{1..4,10,15,18} (7 alike) : Scope
  Scope17 : Scope  NumInputPorts=2
  Sum1 : Sum
  Sum3 : Sum  Inputs=2
  Sum4 : Sum  Inputs=2
  Sum5 : Sum
  Switch{3,5,7..10} (6 alike) : Switch  Criteria=u2 > Threshold  Threshold=0.5  SaturateOnIntegerOverflow=off  InputSameDT=off
  Switch2 : Switch  Criteria=u2 > Threshold  Threshold=10  SaturateOnIntegerOverflow=off  InputSameDT=off
  Switch6 : Switch  Criteria=u2 > Threshold  Threshold=10  SaturateOnIntegerOverflow=off  InputSameDT=off
  Terminator : Terminator
  Terminator1 : Terminator
  Tinitial12 : Constant  Value=1/3600
  on? (I/O)2 : Constant  Value=20  OutDataTypeStr=double
  on? (I/O)9 : Constant  Value=20  OutDataTypeStr=double
  tempout if off : Constant  Value=0
  tempout if on : Constant  Value=0
  Out1 : Outport  VectorParamsAs1DForOutWhenUnconnected=off
  Out2 : Outport  Port=2  VectorParamsAs1DForOutWhenUnconnected=off
  Out3 : Outport  Port=3  VectorParamsAs1DForOutWhenUnconnected=off
  Out4 : Outport  Port=4  VectorParamsAs1DForOutWhenUnconnected=off
  Out5 : Outport  Port=5  VectorParamsAs1DForOutWhenUnconnected=off
  Out6 : Outport  Port=6  VectorParamsAs1DForOutWhenUnconnected=off
  wires:
  Data Type Conversion10/1 -> Switch5/2
  Data Type Conversion2/1 -> Out4/1, Data Type Conversion8/1, HeatPump_Simplified/4(Ctrl)
  Based on 50.35l/s per kW (https://designbuilder.co.uk/helpv5.5/Content/AirToWaterHeatPumpASHPData.htm)1/1 -> Switch9/1
  Massflow when system is off1/1 -> Switch5/3
  [SH] -> Logical Operator1/2
  [N_On] -> Data Type Conversion5/1
  In7/1 -> [SH]
  on? (I/O)9/1 -> Switch6/3
  Bus Selector2/1 -> Sum4/1
  HeatPump_Simplified1/2("T_out ") -> Switch7/1
  Product3/1 -> HeatPump_Simplified/6(mdot_hot), Scope10/1
  [T_Ot] -> HeatPump_Simplified/3(Tamb)
  Discrete-Time Integrator/1 -> Product4/1
  Logical Operator2/1 -> Data Type Conversion3/1
  [D_On] -> Logical Operator2/1
  Data Type Conversion3/1 -> Out3/1, HeatPump_Simplified1/4(Ctrl), Sum5/1
  Bus Selector1/1 -> Sum4/2
  [N_On] -> Product3/2
  HeatPump_Simplified/1(T_source) -> Terminator/1
  Massflow when system is off2/1 -> Switch3/3
  Digital Clock1/1 -> Switch6/2
  tempout if on/1 -> Switch8/3
  Switch2/1 -> HeatPump_Simplified1/2(THB_r)
  [N_On] -> Switch8/2
  HeatPump_Simplified/2("T_out ") -> Switch8/1
  on? (I/O)2/1 -> Switch2/3
  Data Type Conversion6/1 -> Logical Operator3/1
  Logical Operator6/1 -> Data Type Conversion2/1
  Switch10/1 -> Scope15/1, HeatPump_Simplified/5(mdot_cold)
  Switch6/1 -> Scope3/1, Relay2/1, HeatPump_Simplified/2(THB_r)
  Massflow when system is off3/1 -> Switch9/3
  Switch9/1 -> HeatPump_Simplified1/5(mdot_cold)
  Sum5/1 -> Out1/1
  Data Type Conversion5/1 -> Switch10/2
  Switch7/1 -> Sum1/1
  HeatPump_Simplified/5(Main Delta) -> HeatPump_Simplified1/7(Main Delta In)
  tempout if off/1 -> Switch7/3
  HeatPump_Simplified1/1(T_source) -> Terminator1/1
  [SH] -> Logical Operator2/2
  Data Type Conversion4/1 -> Switch3/2
  Data Type Conversion7/1 -> Switch9/2
  [T_Ot] -> HeatPump_Simplified1/3(Tamb)
  Switch5/1 -> Product3/1
  HeatPump_Simplified/4(Real P_Therm) -> Discrete-Time Integrator/1, Sum3/2, Scope18/1
  [D_On] -> Data Type Conversion7/1
  Massflow when system is off4/1 -> Switch10/3
  [MFT] -> Switch5/1
  In1/1 -> [T_Ot]
  Ground1/1 -> Scope17/1
  [MixT] -> Switch2/1
  Switch3/1 -> Scope2/1, HeatPump_Simplified1/6(mdot_hot)
  [MixT] -> Switch6/1
  Based on 50.35l/s per kW (https://designbuilder.co.uk/helpv5.5/Content/AirToWaterHeatPumpASHPData.htm)2/1 -> Switch10/1
  HeatPump_Simplified1/5(Defrost Delta) -> HeatPump_Simplified/7(Defrost Delta In)
  Tinitial12/1 -> Product4/2
  Switch8/1 -> Sum1/2
  [T_Ot] -> HeatPump_Simplified/1(THBsource)
  Product4/1 -> Scope17/2
  Relay2/1 -> Logical Operator6/1
  Data Type Conversion8/1 -> Sum5/2
  [D_On] -> Data Type Conversion6/1
  [D_On] -> Logical Operator1/1
  [SH] -> Logical Operator4/2
  [SH] -> Logical Operator6/4
  HeatPump_Simplified1/4(Real P_Therm) -> Sum3/1
  Logical Operator3/1 -> Switch7/2
  Digital Clock/1 -> Switch2/2
  HeatPump_Simplified/3(HPdat) -> Bus Selector1/1
  HeatPump_Simplified1/3(HPdat) -> Bus Selector2/1
  [GCS] -> Logical Operator6/2
  [T_Ot] -> HeatPump_Simplified1/1(THBsource)
  [MFT] -> Switch3/1
  Logical Operator1/1 -> Data Type Conversion4/1
  [SH] -> Logical Operator3/2
  Logical Operator4/1 -> Data Type Conversion10/1
  [N_On] -> Logical Operator6/3
  [GCS] -> Logical Operator4/1
  Sum4/1 -> Out6/1
  Sum3/1 -> Out5/1
  Sum1/1 -> Scope1/1, Out2/1
  In4/1 -> [MixT]
  In2/1 -> [N_On]
  In3/1 -> [D_On]
  In6/1 -> [GCS]
  In5/1 -> [MFT]
  [N_On] -> Add/2
  Add/1 -> Scope4/1
  [D_On] -> Add/1
  In8/1 -> HeatPump_Simplified/8(Defrost Delta In1)
